simulink model "TEST1_MiniHVAC_Zone"  (R2025b)
settings: Solver=ode3  StartTime=0.0  StopTime=200  FixedStep=0.1  RelTol=1e-3
settings Model: Creator=daniel.camacho  LastModifiedBy=daniel.camacho

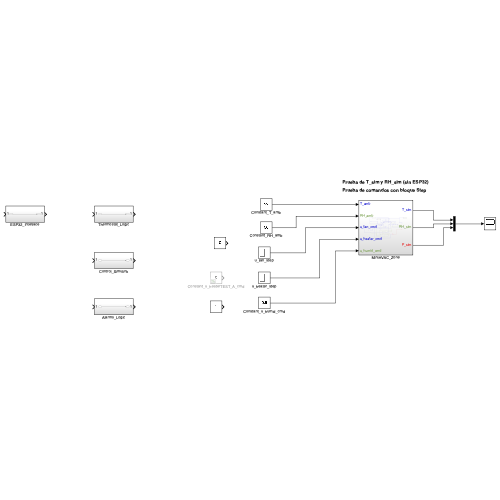
[thumbnail: Simulink's stored preview of the top-level diagram]
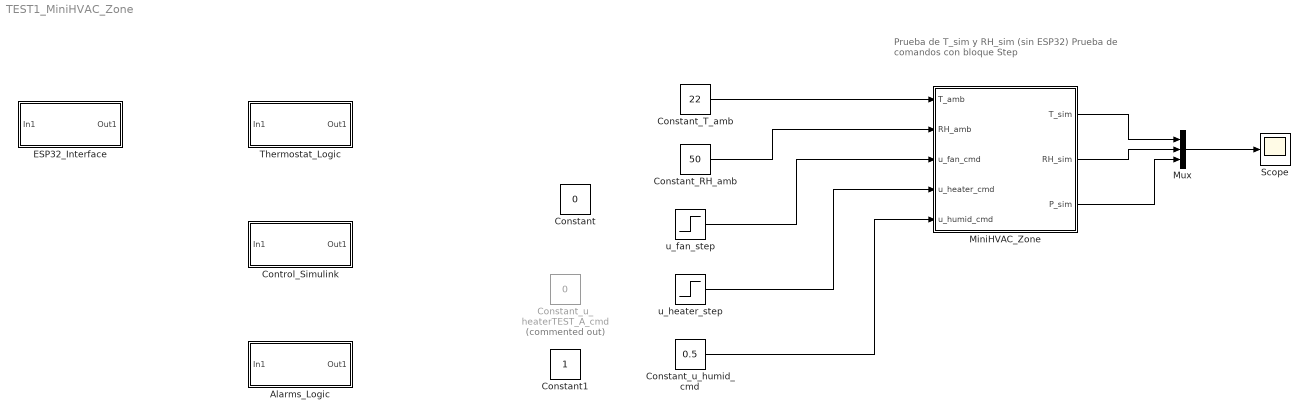
== system TEST1_MiniHVAC_Zone ==
  note: Prueba de T_sim y RH_sim (sin ESP32)
      |
      | Prueba de comandos con bloque Step
  Alarms_Logic : Subsystem
  Constant : Constant  Value=0
  Constant1 : Constant
  Constant_RH_amb : Constant  Value=50
  Constant_T_amb : Constant  Value=22
  Constant_u_heaterTEST_A_cmd : Constant  Commented=on  Value=0
  Constant_u_humid_cmd : Constant  Value=0.5
  Control_Simulink : Subsystem
  ESP32_Interface : Subsystem
  MiniHVAC_Zone : Subsystem
  Mux : Mux  Inputs=3
  Scope : Scope
      settings: ActiveDisplayYMinimum=-21.778332690309028  ActiveDisplayYMaximum=88.0793379212709
  Thermostat_Logic : Subsystem
  u_fan_step : Step  Time=20  SampleTime=0
  u_heater_step : Step  Time=100  SampleTime=0
  wires:
  Constant_T_amb/1 -> MiniHVAC_Zone/1(T_amb)
  Constant_RH_amb/1 -> MiniHVAC_Zone/2(RH_amb)
  MiniHVAC_Zone/1(T_sim) -> Mux/1
  MiniHVAC_Zone/2(RH_sim) -> Mux/2
  Mux/1 -> Scope/1
  MiniHVAC_Zone/3(P_sim) -> Mux/3
  Constant_u_humid_cmd/1 -> MiniHVAC_Zone/5(u_humid_cmd)
  u_fan_step/1 -> MiniHVAC_Zone/3(u_fan_cmd)
  u_heater_step/1 -> MiniHVAC_Zone/4(u_heater_cmd)

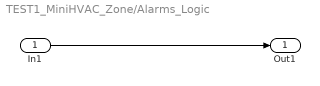
== system TEST1_MiniHVAC_Zone/Alarms_Logic ==
  In1 : Inport
  Out1 : Outport
  wires:
  In1/1 -> Out1/1

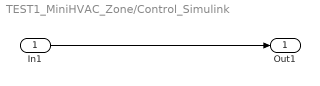
== system TEST1_MiniHVAC_Zone/Control_Simulink ==
  In1 : Inport
  Out1 : Outport
  wires:
  In1/1 -> Out1/1

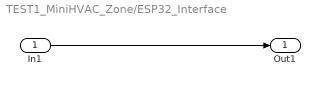
== system TEST1_MiniHVAC_Zone/ESP32_Interface ==
  In1 : Inport
  Out1 : Outport
  wires:
  In1/1 -> Out1/1

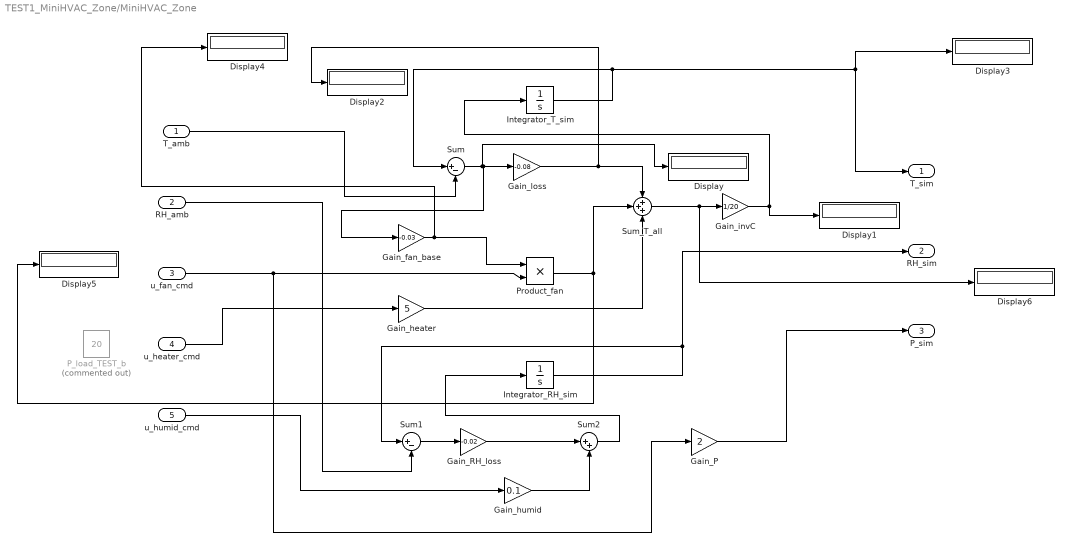
== system TEST1_MiniHVAC_Zone/MiniHVAC_Zone ==
  T_amb : Inport
  RH_amb : Inport  Port=2
  u_fan_cmd : Inport  Port=3
  u_heater_cmd : Inport  Port=4
  u_humid_cmd : Inport  Port=5
  Display{,1..6} (7 alike) : Display
  Gain_P : Gain  Gain=2
  Gain_RH_loss : Gain  Gain=-0.02
  Gain_fan_base : Gain  Gain=-0.03
  Gain_heater : Gain  Gain=5
  Gain_humid : Gain  Gain=0.1
  Gain_invC : Gain  Gain=1/20
  Gain_loss : Gain  Gain=-0.08
  Integrator_RH_sim : Integrator  InitialCondition=40
  Integrator_T_sim : Integrator  InitialCondition=22
  P_load_TEST_b : Constant  Commented=on  Value=20
  Product_fan : Product
  Sum : Sum  Inputs=|+-
  Sum1 : Sum  Inputs=|+-
  Sum2 : Sum  Inputs=|++
  Sum_T_all : Sum  Inputs=+++
  T_sim : Outport
  RH_sim : Outport  Port=2
  P_sim : Outport  Port=3
  wires:
  Integrator_T_sim/1 -> Sum/1, T_sim/1, Display3/1
  T_amb/1 -> Sum/2
  Gain_fan_base/1 -> Product_fan/1, Display4/1
  u_fan_cmd/1 -> Gain_P/1, Product_fan/2
  u_heater_cmd/1 -> Gain_heater/1
  Sum/1 -> Display/1, Gain_fan_base/1, Gain_loss/1
  Gain_loss/1 -> Display2/1, Sum_T_all/1
  Product_fan/1 -> Sum_T_all/2, Display5/1
  Gain_heater/1 -> Sum_T_all/3
  Sum_T_all/1 -> Display6/1, Gain_invC/1
  Gain_invC/1 -> Integrator_T_sim/1, Display1/1
  Integrator_RH_sim/1 -> RH_sim/1, Sum1/1
  RH_amb/1 -> Sum1/2
  Sum1/1 -> Gain_RH_loss/1
  u_humid_cmd/1 -> Gain_humid/1
  Gain_RH_loss/1 -> Sum2/1
  Gain_humid/1 -> Sum2/2
  Sum2/1 -> Integrator_RH_sim/1
  Gain_P/1 -> P_sim/1

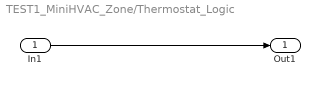
== system TEST1_MiniHVAC_Zone/Thermostat_Logic ==
  In1 : Inport
  Out1 : Outport
  wires:
  In1/1 -> Out1/1
